simulink subsystem "Sub_Plant_and_Environment_Model"  (R2020a)
settings: Solver=VariableStepAuto  StartTime=0.0  StopTime=10.0  RelTol=1e-3
values from neighbouring files (symbols this model uses):
  a_rad = deg2rad(a)    [plant_init.m]
  AF = [0.12, 0.22, 0.292]    [plant_init.m]
  l1 = [(D14(3)-RB(3)+PZ(1)*dz),     (D14(3)-RB(3)+PZ(1)*dz),     -hypot( D14(1)-RB(1), D14(2)-RB(2))]    [plant_init.m]
  l2 = [-(D14(3)-RB(3)+PZ(2)*dz),      (D14(3)-RB(3)+PZ(2)*dz),      -hypot( D14(1)+RB(1), D14(2)-RB(2))]    [plant_init.m]
  l3 = [(D14(3)-RB(3)+PZ(3)*dz),      (D14(3)-RB(3)+PZ(3)*dz),      hypot(D14(1)+RB(1), D14(2)+RB(2))]    [plant_init.m]
  l4 = [-(D14(3)-RB(3)+PZ(4)*dz),      (D14(3)-RB(3)+PZ(4)*dz),      hypot(D14(1)-RB(1), D14(2)+RB(2))]    [plant_init.m]
  l5 = [(D58(2)-RB(2)+PZ(1)*dz),      -(D58(1)-RB(1)+PZ(1)*dz), 0]    [plant_init.m]
  l6 = [-(D58(2)-RB(2)+PZ(2)*dz),       -(D58(1)+RB(1)+PZ(2)*dz), 0]    [plant_init.m]
  l7 = [-(D58(2)+RB(2)+PZ(3)*dz),     (D58(1)+RB(1)+PZ(3)*dz), 0]    [plant_init.m]
  l8 = [(D58(2)+RB(2)+PZ(4)*dz),      (D58(1)-RB(1)+PZ(2)*dz), 0]    [plant_init.m]
  mass = 33.95    [plant_init.m]
  N = T200Spec16V{:,6}    [InitController.m]    (also in plant_init.m)
  PWM = T200Spec16V{:,1}    [InitController.m]    (also in plant_init.m)
  RB = [ 0.001,      -0.003,       0.027]    [plant_init.m]
  RG = [ 0.001,      -0.003,       0.027]    [plant_init.m]
  rho = 998    [plant_init.m]
  volume = 0.027    [plant_init.m]
libraries: sharedtransform x11, vrlib x9, shared6dof x1, aerolibasang x1
(part 2 of 2)

== system Sub_Plant_and_Environment_Model/Propulsion Forces & Moments/Force and moments due to Thrust/Thrust to Propulsion /Moment computation/Moment Moteur 7 ==
  Thrust : Inport
  Constant : Constant  Value=[a;b;c]
  Cross Product : vrlib/Utilities/Cross Product
  Moment : Outport  VectorParamsAs1DForOutWhenUnconnected=off
  wires:
  Cross Product/1 -> Moment/1
  Thrust/1 -> Cross Product/2
  Constant/1 -> Cross Product/1

== system Sub_Plant_and_Environment_Model/Propulsion Forces & Moments/Force and moments due to Thrust/Thrust to Propulsion /Moment computation/Moment Moteur 8 ==
  Thrust : Inport
  Constant : Constant  Value=[a;b;c]
  Cross Product : vrlib/Utilities/Cross Product
  Moment : Outport  VectorParamsAs1DForOutWhenUnconnected=off
  wires:
  Cross Product/1 -> Moment/1
  Thrust/1 -> Cross Product/2
  Constant/1 -> Cross Product/1

== matlab function Sub_Plant_and_Environment_Model/Environmental Forces & Moments/Hydrodynamic Forces/Hydrodynamic Forces - Accurate/Force Exerted due to Lift (Body Axis)/MATLAB Function ==
  data: u input; y output
function y = fcn(u)
if u>pi/2
    u = u-pi;
elseif u < -pi/2
    u = u + pi;
end

y = 1 * (u) + 0;

== matlab function Sub_Plant_and_Environment_Model/Propulsion Forces & Moments/Input commands to Thrust/PWM Signals to Thrust /MATLAB Function ==
  data: u input; y output
function y = Normalize(u)
y = (u-1500)*150/400;

== matlab function Sub_Plant_and_Environment_Model/Propulsion Forces & Moments/Input commands to Thrust/PWM Signals to Thrust /MATLAB Function1 ==
  data: u input; y output
function y = Normalize(u)
y = (u-1500)*150/400;

== matlab function Sub_Plant_and_Environment_Model/Propulsion Forces & Moments/Input commands to Thrust/PWM Signals to Thrust /MATLAB Function2 ==
  data: u input; y output
function y = Normalize(u)
y = (u-1500)*150/400;

== matlab function Sub_Plant_and_Environment_Model/Propulsion Forces & Moments/Input commands to Thrust/PWM Signals to Thrust /MATLAB Function3 ==
  data: u input; y output
function y = Normalize(u)
y = (u-1500)*150/400;

== matlab function Sub_Plant_and_Environment_Model/Propulsion Forces & Moments/Input commands to Thrust/PWM Signals to Thrust /MATLAB Function4 ==
  data: u input; y output
function y = Normalize(u)
y = (u-1500)*150/400;

== matlab function Sub_Plant_and_Environment_Model/Dynamics solver/Post-Processing/MATLAB Function ==
  data: Position input; srf_in input
function Visualize(Position, srf_in)

    coder.extrinsic('setax'); 
    setax(Position, srf_in);  

end

== matlab function Sub_Plant_and_Environment_Model/Propulsion Forces & Moments/Input commands to Thrust/PWM Signals to Thrust /MATLAB Function5 ==
  data: u input; y output
function y = Normalize(u)
y = (u-1500)*150/400;

== matlab function Sub_Plant_and_Environment_Model/Propulsion Forces & Moments/Input commands to Thrust/PWM Signals to Thrust /MATLAB Function6 ==
  data: u input; y output
function y = Normalize(u)
y = (u-1500)*150/400;

== matlab function Sub_Plant_and_Environment_Model/Propulsion Forces & Moments/Input commands to Thrust/PWM Signals to Thrust /MATLAB Function7 ==
  data: u input; y output
function y = Normalize(u)
y = (u-1500)*150/400;

== matlab function Sub_Plant_and_Environment_Model/Environmental Forces & Moments/Hydrodynamic Forces/Hydrodynamic Forces - Accurate/Force Exerted due to Drag (Body Axis)/MATLAB Function ==
  data: u input; C_D output
function C_D = Calculate_Drag_Coeff(u)
if u>pi/2
    u = u-pi;
elseif u < -pi/2
    u = u + pi;
end
C_D = 5.25*(u.^2) - 0.315 * (u) + 0.732;
